simulink model "equivalent"  (R2018a)
settings: Solver=VariableStepAuto  StartTime=0.0  StopTime=10.0  RelTol=1e-3
undefined symbols (not defined in the file): DiscIntNeverNeededParam, sigbuilder_block
libraries: simulink x479
(part 4 of 10)

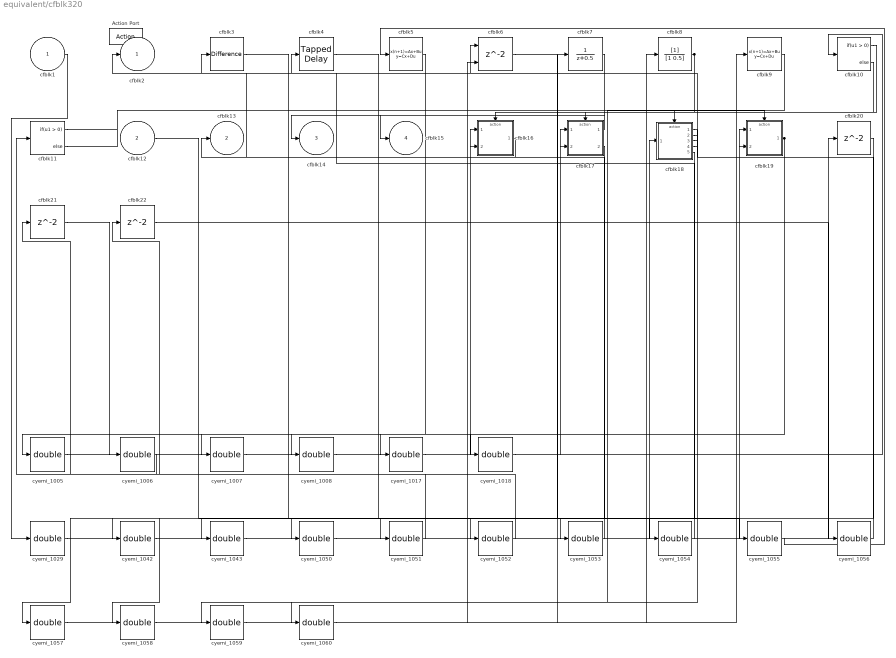
== system equivalent/cfblk320 ==
  cfblk1 : Inport
  cfblk12 : Inport  Port=2
  Action Port : ActionPort  ActionType=else
  cfblk10 : If  SampleTime=1
  cfblk11 : If  SampleTime=1
  cfblk16 : Subsystem  TreatAsAtomicUnit=on
  cfblk17 : Subsystem  TreatAsAtomicUnit=on
  cfblk18 : Subsystem  TreatAsAtomicUnit=on
  cfblk19 : Subsystem  TreatAsAtomicUnit=on
  cfblk20 : Delay
  cfblk21 : Delay
  cfblk22 : Delay
  cfblk3 : simulink/Discrete/Difference  ICPrevInput=0.0  OutMin=[]  OutMax=[]  OutDataTypeStr=Inherit: Inherit via back propagation  OutDataType=fixdt(1, 16)  OutScaling=2^-10  DoSatur=off
  cfblk4 : simulink/Discrete/Tapped Delay  vinit=0.0  samptime=-1  NumDelays=1  DelayOrder=Oldest  includeCurrent=off
  cfblk5 : DiscreteStateSpace  SampleTime=-1
  cfblk6 : Delay  ShowEnablePort=on
      settings: InputPortMap=u0,e6
  cfblk7 : DiscreteTransferFcn
  cfblk8 : DiscreteFilter
  cfblk9 : DiscreteStateSpace  SampleTime=-1
  cyemi_{1005..1008,1017..1018,1029,1042..1043,1050..1060} (20 alike) : DataTypeConversion  OutDataTypeStr=double
  cfblk2 : Outport
  cfblk13 : Outport  Port=2
  cfblk14 : Outport  Port=3
  cfblk15 : Outport  Port=4
  wires:
  cfblk8/1 -> cyemi_1007/1, cyemi_1050/1, cyemi_1060/1
  cfblk16/1(cfblk2) -> cfblk13/1
  cfblk19/1(cfblk2) -> cyemi_1005/1, cyemi_1008/1
  cfblk17/1(cfblk2) -> cfblk14/1
  cfblk18/3(cfblk14) -> cfblk2/1
  cfblk7/1 -> cfblk15/1
  cfblk10/1 -> cfblk16/Action
  cfblk10/2 -> cfblk17/Action
  cfblk11/1 -> cfblk18/Action
  cfblk11/2 -> cfblk19/Action
  cyemi_1005/1 -> cfblk10/1
  cyemi_1006/1 -> cfblk11/1
  cfblk21/1 -> cyemi_1006/1
  cyemi_1007/1 -> cfblk16/1(cfblk1)
  cyemi_1008/1 -> cfblk16/2(cfblk8)
  cyemi_1017/1 -> cfblk17/1(cfblk1)
  cfblk5/1 -> cyemi_1017/1
  cyemi_1018/1 -> cfblk17/2(cfblk10)
  cfblk18/1(cfblk2) -> cyemi_1018/1
  cyemi_1029/1 -> cfblk18/1(cfblk1)
  cfblk1/1 -> cyemi_1029/1
  cyemi_1042/1 -> cfblk19/1(cfblk1)
  cfblk20/1 -> cyemi_1042/1
  cyemi_1043/1 -> cfblk19/2(cfblk8)
  cfblk18/2(cfblk13) -> cyemi_1043/1
  cyemi_1050/1 -> cfblk20/1
  cyemi_1051/1 -> cfblk21/1
  cfblk3/1 -> cyemi_1051/1
  cyemi_1052/1 -> cfblk22/1
  cfblk4/1 -> cyemi_1052/1
  cyemi_1053/1 -> cfblk3/1
  cfblk9/1 -> cyemi_1053/1
  cyemi_1054/1 -> cfblk4/1
  cfblk6/1 -> cyemi_1054/1
  cyemi_1055/1 -> cfblk5/1
  cfblk12/1 -> cyemi_1055/1
  cyemi_1056/1 -> cfblk6/1
  cfblk22/1 -> cyemi_1056/1
  cyemi_1057/1 -> cfblk6/2
  cfblk18/5(cfblk16) -> cyemi_1057/1
  cyemi_1058/1 -> cfblk7/1
  cfblk17/2(cfblk11) -> cyemi_1058/1
  cyemi_1059/1 -> cfblk8/1
  cfblk18/4(cfblk15) -> cyemi_1059/1
  cyemi_1060/1 -> cfblk9/1

== system equivalent/cfblk321 ==
  cfblk1 : Inport
  cfblk6 : Inport  Port=2
  Action Port : ActionPort  ActionType=then
  cfblk10 : Subsystem  TreatAsAtomicUnit=on
  cfblk11 : Delay
  cfblk12 : Delay
  cfblk3 : simulink/Discrete/Transfer Fcn Real Zero  ZeroZ=0.75  ICPrevInput=0.0  DoSatur=off
      settings: SourceProductName=Simulink  SourceProductBaseCode=SL
  cfblk4 : simulink/Discrete/Transfer Fcn Lead or Lag  PoleZ=0.95  ZeroZ=0.75  ICPrevOutput=0.0  ICPrevInput=0.0  DoSatur=off
      settings: SourceProductName=Simulink  SourceProductBaseCode=SL
  cfblk5 : If  SampleTime=1
  cfblk9 : Subsystem  TreatAsAtomicUnit=on
  cyemi_{1063..1064,1075..1081} (9 alike) : DataTypeConversion  OutDataTypeStr=double
  cfblk2 : Outport
  cfblk7 : Outport  Port=2
  cfblk8 : Outport  Port=3
  wires:
  cfblk9/1(cfblk2) -> cfblk8/1, cyemi_1075/1, cyemi_1077/1
  cfblk10/3(cfblk14) -> cfblk7/1
  cfblk3/1 -> cfblk2/1
  cfblk5/1 -> cfblk9/Action
  cfblk5/2 -> cfblk10/Action
  cyemi_1063/1 -> cfblk10/1(cfblk1)
  cfblk11/1 -> cyemi_1063/1
  cyemi_1064/1 -> cfblk10/2(cfblk12)
  cfblk1/1 -> cyemi_1064/1
  cyemi_1075/1 -> cfblk11/1
  cyemi_1076/1 -> cfblk12/1
  cfblk4/1 -> cyemi_1076/1
  cyemi_1077/1 -> cfblk3/1
  cyemi_1078/1 -> cfblk4/1
  cfblk10/2(cfblk13) -> cyemi_1078/1
  cyemi_1079/1 -> cfblk5/1
  cfblk6/1 -> cyemi_1079/1
  cyemi_1080/1 -> cfblk9/1(cfblk1)
  cfblk12/1 -> cyemi_1080/1
  cyemi_1081/1 -> cfblk9/2(cfblk8)
  cfblk10/1(cfblk2) -> cyemi_1081/1

== system equivalent/cfblk322 ==
  cfblk1 : Inport
  cfblk11 : Inport  Port=2
  Action Port : ActionPort  ActionType=else
  cfblk{6,10,13..15} (5 alike) : Delay
  cfblk3 : UnitDelay  SampleTime=-1
  cfblk4 : simulink/Continuous/PID Controller (2DOF)  Controller=PID  TimeDomain=Discrete-time  SampleTime=-1  IntegratorMethod=Forward Euler  FilterMethod=Forward Euler  Form=Parallel  UseFilter=on  ControllerParametersSource=internal  P=1  I=1  D=0  N=100  b=1  c=1  InitialConditionSource=internal  InitialConditionForIntegrator=0  InitialConditionForFilter=0  ExternalReset=none  LimitOutput=off  UpperSaturationLimit=inf  LowerSaturationLimit=-inf  LinearizeAsGain=off  AntiWindupMode=none  Kb=1  TrackingMode=off  Kt=1  PParamMin=[]  PParamMax=[]  IParamMin=[]  IParamMax=[]  DParamMin=[]  DParamMax=[]  NParamMin=[]  NParamMax=[]  bParamMin=[]  bParamMax=[]  cParamMin=[]  cParamMax=[]  KbParamMin=[]  KbParamMax=[]  KtParamMin=[]  KtParamMax=[]  POutMin=[]  POutMax=[]  IOutMin=[]  IOutMax=[]  DOutMin=[]  DOutMax=[]  NOutMin=[]  NOutMax=[]  bOutMin=[]  bOutMax=[]  cOutMin=[]  cOutMax=[]  KbOutMin=[]  KbOutMax=[]  KtOutMin=[]  KtOutMax=[]  IntegratorOutMin=[]  IntegratorOutMax=[]  FilterOutMin=[]  FilterOutMax=[]  SumOutMin=[]  SumOutMax=[]  Sum1OutMin=[]  Sum1OutMax=[]  Sum2OutMin=[]  Sum2OutMax=[]  Sum3OutMin=[]  Sum3OutMax=[]  SumI1OutMin=[]  SumI1OutMax=[]  SumI2OutMin=[]  SumI2OutMax=[]  SumI3OutMin=[]  SumI3OutMax=[]  SumDOutMin=[]  SumDOutMax=[]  SaturationOutMin=[]  SaturationOutMax=[]  IntegratorContinuousStateAttributes=''  IntegratorStateMustResolveToSignalObject=off  IntegratorRTWStateStorageClass=Auto  FilterContinuousStateAttributes=''  FilterStateMustResolveToSignalObject=off  FilterRTWStateStorageClass=Auto  DifferentiatorICPrevScaledInput=0  DifferentiatorOutMin=[]  DifferentiatorOutMax=[]  FilterDiffOutCoefMin=[]  FilterDiffOutCoefMax=[]  SumDenOutMin=[]  SumDenOutMax=[]  SumNumOutMin=[]  SumNumOutMax=[]  ReciprocalOutMin=[]  ReciprocalOutMax=[]  DivideOutMin=[]  DivideOutMax=[]  TunerSelectOption=Transfer Function Based (PID Tuner App)
  cfblk5 : DiscreteZeroPole  Poles=[0 0.5]  Gain=1  SampleTime=-1
  cfblk7 : Delay  DelayLengthSource=Input port
      settings: InputPortMap=u0,p1
  cfblk8 : DiscreteTransferFcn
  cfblk9 : DiscreteZeroPole  Poles=[0 0.5]  Gain=1  SampleTime=-1
  cyemi_{1090..1102} (13 alike) : DataTypeConversion  OutDataTypeStr=double
  cfblk2 : Outport
  cfblk12 : Outport  Port=2
  wires:
  cfblk3/1 -> cfblk2/1
  cfblk8/1 -> cfblk12/1, cyemi_1100/1
  cfblk9/1 -> cyemi_1091/1, cyemi_1098/1
  cyemi_1090/1 -> cfblk10/1
  cfblk6/1 -> cyemi_1090/1
  cyemi_1091/1 -> cfblk13/1
  cyemi_1092/1 -> cfblk14/1
  cfblk10/1 -> cyemi_1092/1
  cyemi_1093/1 -> cfblk15/1
  cfblk7/1 -> cyemi_1093/1
  cyemi_1094/1 -> cfblk3/1
  cfblk1/1 -> cyemi_1094/1
  cyemi_1095/1 -> cfblk4/1
  cfblk13/1 -> cyemi_1095/1
  cyemi_1096/1 -> cfblk4/2
  cfblk14/1 -> cyemi_1096/1
  cyemi_1097/1 -> cfblk5/1
  cfblk15/1 -> cyemi_1097/1
  cyemi_1098/1 -> cfblk6/1
  cyemi_1099/1 -> cfblk7/1
  cfblk11/1 -> cyemi_1099/1
  cyemi_1100/1 -> cfblk7/2
  cyemi_1101/1 -> cfblk8/1
  cfblk5/1 -> cyemi_1101/1
  cyemi_1102/1 -> cfblk9/1
  cfblk4/1 -> cyemi_1102/1

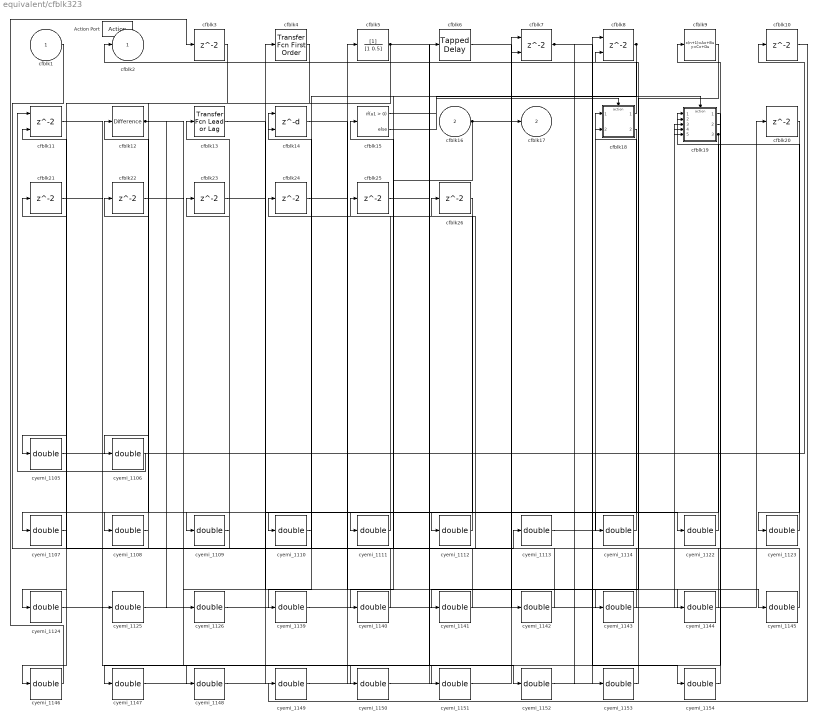
== system equivalent/cfblk323 ==
  cfblk1 : Inport
  cfblk16 : Inport  Port=2
  Action Port : ActionPort  ActionType=then
  cfblk{3,10,20..26} (9 alike) : Delay
  cfblk11 : Delay  ShowEnablePort=on
      settings: InputPortMap=u0,e6
  cfblk12 : simulink/Discrete/Difference  ICPrevInput=0.0  OutMin=[]  OutMax=[]  OutDataTypeStr=Inherit: Inherit via back propagation  OutDataType=fixdt(1, 16)  OutScaling=2^-10  DoSatur=off
  cfblk13 : simulink/Discrete/Transfer Fcn Lead or Lag  PoleZ=0.95  ZeroZ=0.75  ICPrevOutput=0.0  ICPrevInput=0.0  DoSatur=off
      settings: SourceProductName=Simulink  SourceProductBaseCode=SL
  cfblk14 : Delay  DelayLengthSource=Input port
      settings: InputPortMap=u0,p1
  cfblk15 : If  SampleTime=1
  cfblk18 : Subsystem  TreatAsAtomicUnit=on
  cfblk19 : Subsystem  TreatAsAtomicUnit=on
  cfblk4 : simulink/Discrete/Transfer Fcn First Order  PoleZ=0.95  ICPrevOutput=0.0  DoSatur=off
      settings: SourceProductName=Simulink
  cfblk5 : DiscreteFilter
  cfblk6 : simulink/Discrete/Tapped Delay  vinit=0.0  samptime=-1  NumDelays=1  DelayOrder=Oldest  includeCurrent=off
  cfblk7 : Delay  ShowEnablePort=on
      settings: InputPortMap=u0,e6
  cfblk8 : Delay  ShowEnablePort=on
      settings: InputPortMap=u0,e6
  cfblk9 : DiscreteStateSpace  SampleTime=-1
  cyemi_{1105..1114,1122..1126,1139..1154} (31 alike) : DataTypeConversion  OutDataTypeStr=double
  cfblk2 : Outport
  cfblk17 : Outport  Port=2
  wires:
  cfblk16/1 -> cfblk17/1, cyemi_1111/1
  cfblk5/1 -> cyemi_1107/1, cyemi_1152/1
  cfblk12/1 -> cyemi_1106/1, cyemi_1126/1, cyemi_1145/1
  cfblk18/1(cfblk2) -> cfblk2/1
  cfblk8/1 -> cyemi_1139/1, cyemi_1140/1
  cfblk7/1 -> cyemi_1153/1, cyemi_1154/1
  cfblk19/3(cfblk16) -> cyemi_1109/1, cyemi_1110/1
  cfblk15/1 -> cfblk18/Action
  cfblk15/2 -> cfblk19/Action
  cyemi_1105/1 -> cfblk10/1
  cfblk4/1 -> cyemi_1105/1
  cyemi_1106/1 -> cfblk11/1
  cyemi_1107/1 -> cfblk11/2
  cyemi_1108/1 -> cfblk12/1
  cfblk3/1 -> cyemi_1108/1
  cyemi_1109/1 -> cfblk13/1
  cyemi_1110/1 -> cfblk14/1
  cyemi_1111/1 -> cfblk14/2
  cyemi_1112/1 -> cfblk15/1
  cfblk23/1 -> cyemi_1112/1
  cyemi_1113/1 -> cfblk18/1(cfblk1)
  cfblk1/1 -> cyemi_1113/1
  cyemi_1114/1 -> cfblk18/2(cfblk9)
  cfblk25/1 -> cyemi_1114/1
  cyemi_1122/1 -> cfblk19/1(cfblk1)
  cfblk24/1 -> cyemi_1122/1
  cyemi_1123/1 -> cfblk19/2(cfblk11)
  cfblk20/1 -> cyemi_1123/1
  cyemi_1124/1 -> cfblk19/3(cfblk12)
  cfblk18/2(cfblk10) -> cyemi_1124/1
  cyemi_1125/1 -> cfblk19/4(cfblk13)
  cfblk21/1 -> cyemi_1125/1
  cyemi_1126/1 -> cfblk19/5(cfblk14)
  cyemi_1139/1 -> cfblk20/1
  cyemi_1140/1 -> cfblk21/1
  cyemi_1141/1 -> cfblk22/1
  cfblk9/1 -> cyemi_1141/1
  cyemi_1142/1 -> cfblk23/1
  cfblk6/1 -> cyemi_1142/1
  cyemi_1143/1 -> cfblk24/1
  cfblk14/1 -> cyemi_1143/1
  cyemi_1144/1 -> cfblk25/1
  cfblk13/1 -> cyemi_1144/1
  cyemi_1145/1 -> cfblk26/1
  cyemi_1146/1 -> cfblk3/1
  cfblk26/1 -> cyemi_1146/1
  cyemi_1147/1 -> cfblk4/1
  cfblk19/2(cfblk15) -> cyemi_1147/1
  cyemi_1148/1 -> cfblk5/1
  cfblk19/1(cfblk2) -> cyemi_1148/1
  cyemi_1149/1 -> cfblk6/1
  cfblk10/1 -> cyemi_1149/1
  cyemi_1150/1 -> cfblk7/1
  cfblk11/1 -> cyemi_1150/1
  cyemi_1151/1 -> cfblk7/2
  cfblk22/1 -> cyemi_1151/1
  cyemi_1152/1 -> cfblk8/1
  cyemi_1153/1 -> cfblk8/2
  cyemi_1154/1 -> cfblk9/1

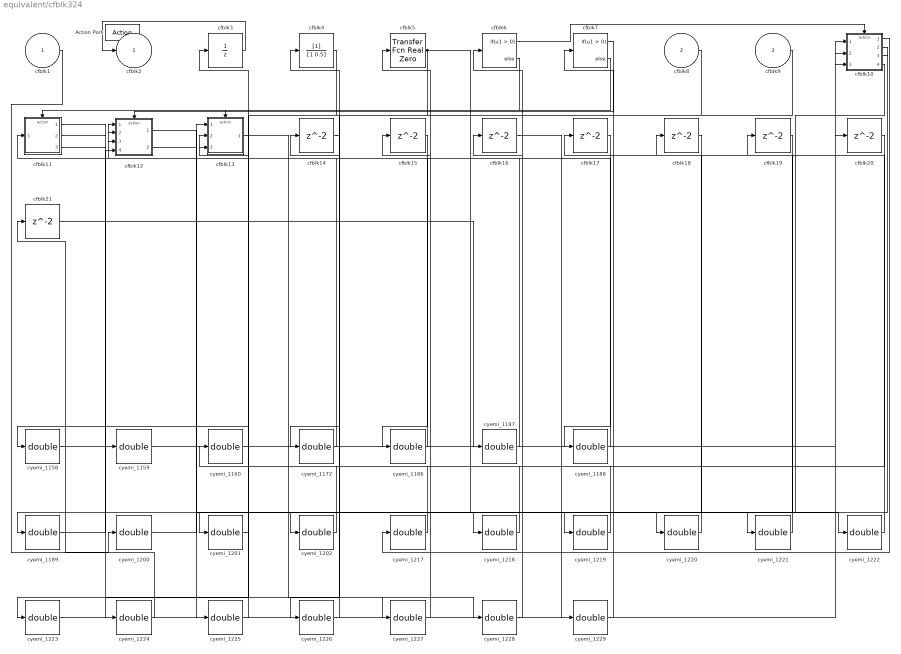
== system equivalent/cfblk324 ==
  cfblk1 : Inport
  cfblk8 : Inport  Port=2
  cfblk9 : Inport  Port=3
  Action Port : ActionPort  ActionType=else
  cfblk10 : Subsystem  TreatAsAtomicUnit=on
  cfblk11 : Subsystem  TreatAsAtomicUnit=on
  cfblk12 : Subsystem  TreatAsAtomicUnit=on
  cfblk13 : Subsystem  TreatAsAtomicUnit=on
  cfblk{14..21} (8 alike) : Delay
  cfblk3 : UnitDelay  SampleTime=-1
  cfblk4 : DiscreteFilter
  cfblk5 : simulink/Discrete/Transfer Fcn Real Zero  ZeroZ=0.75  ICPrevInput=0.0  DoSatur=off
      settings: SourceProductName=Simulink  SourceProductBaseCode=SL
  cfblk6 : If  SampleTime=1
  cfblk7 : If  SampleTime=1
  cyemi_{1158..1160,1172,1186..1189,1200..1202,1217..1229} (24 alike) : DataTypeConversion  OutDataTypeStr=double
  cfblk2 : Outport
  wires:
  cfblk3/1 -> cfblk2/1
  cfblk5/1 -> cyemi_1222/1, cyemi_1223/1
  cfblk6/1 -> cfblk10/Action
  cfblk6/2 -> cfblk11/Action
  cfblk7/1 -> cfblk12/Action
  cfblk7/2 -> cfblk13/Action
  cyemi_1158/1 -> cfblk10/1(cfblk1)
  cfblk4/1 -> cyemi_1158/1
  cyemi_1159/1 -> cfblk10/2(cfblk12)
  cfblk11/2(cfblk10) -> cyemi_1159/1
  cyemi_1160/1 -> cfblk10/3(cfblk13)
  cfblk20/1 -> cyemi_1160/1
  cyemi_1172/1 -> cfblk11/1(cfblk1)
  cfblk9/1 -> cyemi_1172/1
  cyemi_1186/1 -> cfblk12/1(cfblk1)
  cfblk15/1 -> cyemi_1186/1
  cyemi_1187/1 -> cfblk12/2(cfblk12)
  cfblk21/1 -> cyemi_1187/1
  cyemi_1188/1 -> cfblk12/3(cfblk13)
  cfblk17/1 -> cyemi_1188/1
  cyemi_1189/1 -> cfblk12/4(cfblk14)
  cfblk18/1 -> cyemi_1189/1
  cyemi_1200/1 -> cfblk13/1(cfblk1)
  cfblk1/1 -> cyemi_1200/1
  cyemi_1201/1 -> cfblk13/2(cfblk13)
  cfblk19/1 -> cyemi_1201/1
  cyemi_1202/1 -> cfblk13/3(cfblk14)
  cfblk14/1 -> cyemi_1202/1
  cyemi_1217/1 -> cfblk14/1
  cfblk10/1(cfblk2) -> cyemi_1217/1
  cyemi_1218/1 -> cfblk15/1
  cfblk10/2(cfblk14) -> cyemi_1218/1
  cyemi_1219/1 -> cfblk16/1
  cfblk12/1(cfblk2) -> cyemi_1219/1
  cyemi_1220/1 -> cfblk17/1
  cfblk10/3(cfblk15) -> cyemi_1220/1
  cyemi_1221/1 -> cfblk18/1
  cfblk10/4(cfblk16) -> cyemi_1221/1
  cyemi_1222/1 -> cfblk19/1
  cyemi_1223/1 -> cfblk20/1
  cyemi_1224/1 -> cfblk21/1
  cfblk11/3(cfblk11) -> cyemi_1224/1
  cyemi_1225/1 -> cfblk3/1
  cfblk12/2(cfblk15) -> cyemi_1225/1
  cyemi_1226/1 -> cfblk4/1
  cfblk8/1 -> cyemi_1226/1
  cyemi_1227/1 -> cfblk5/1
  cfblk11/1(cfblk2) -> cyemi_1227/1
  cyemi_1228/1 -> cfblk6/1
  cfblk13/1(cfblk2) -> cyemi_1228/1
  cyemi_1229/1 -> cfblk7/1
  cfblk16/1 -> cyemi_1229/1

== system equivalent/cfblk325 ==
  cfblk1 : Inport
  cfblk6 : Inport  Port=2
  Action Port : ActionPort  ActionType=then
  cfblk3 : Delay
  cfblk4 : simulink/Continuous/PID Controller (2DOF)  Controller=PID  TimeDomain=Discrete-time  SampleTime=-1  IntegratorMethod=Forward Euler  FilterMethod=Forward Euler  Form=Parallel  UseFilter=on  ControllerParametersSource=internal  P=1  I=1  D=0  N=100  b=1  c=1  InitialConditionSource=internal  InitialConditionForIntegrator=0  InitialConditionForFilter=0  ExternalReset=none  LimitOutput=off  UpperSaturationLimit=inf  LowerSaturationLimit=-inf  LinearizeAsGain=off  AntiWindupMode=none  Kb=1  TrackingMode=off  Kt=1  PParamMin=[]  PParamMax=[]  IParamMin=[]  IParamMax=[]  DParamMin=[]  DParamMax=[]  NParamMin=[]  NParamMax=[]  bParamMin=[]  bParamMax=[]  cParamMin=[]  cParamMax=[]  KbParamMin=[]  KbParamMax=[]  KtParamMin=[]  KtParamMax=[]  POutMin=[]  POutMax=[]  IOutMin=[]  IOutMax=[]  DOutMin=[]  DOutMax=[]  NOutMin=[]  NOutMax=[]  bOutMin=[]  bOutMax=[]  cOutMin=[]  cOutMax=[]  KbOutMin=[]  KbOutMax=[]  KtOutMin=[]  KtOutMax=[]  IntegratorOutMin=[]  IntegratorOutMax=[]  FilterOutMin=[]  FilterOutMax=[]  SumOutMin=[]  SumOutMax=[]  Sum1OutMin=[]  Sum1OutMax=[]  Sum2OutMin=[]  Sum2OutMax=[]  Sum3OutMin=[]  Sum3OutMax=[]  SumI1OutMin=[]  SumI1OutMax=[]  SumI2OutMin=[]  SumI2OutMax=[]  SumI3OutMin=[]  SumI3OutMax=[]  SumDOutMin=[]  SumDOutMax=[]  SaturationOutMin=[]  SaturationOutMax=[]  IntegratorContinuousStateAttributes=''  IntegratorStateMustResolveToSignalObject=off  IntegratorRTWStateStorageClass=Auto  FilterContinuousStateAttributes=''  FilterStateMustResolveToSignalObject=off  FilterRTWStateStorageClass=Auto  DifferentiatorICPrevScaledInput=0  DifferentiatorOutMin=[]  DifferentiatorOutMax=[]  FilterDiffOutCoefMin=[]  FilterDiffOutCoefMax=[]  SumDenOutMin=[]  SumDenOutMax=[]  SumNumOutMin=[]  SumNumOutMax=[]  ReciprocalOutMin=[]  ReciprocalOutMax=[]  DivideOutMin=[]  DivideOutMax=[]  TunerSelectOption=Transfer Function Based (PID Tuner App)
  cfblk5 : simulink/Discrete/Tapped Delay  vinit=0.0  samptime=-1  NumDelays=1  DelayOrder=Oldest  includeCurrent=off
  cyemi_{1232..1235} (4 alike) : DataTypeConversion  OutDataTypeStr=double
  cfblk2 : Outport
  cfblk7 : Outport  Port=2
  wires:
  cfblk3/1 -> cfblk2/1, cyemi_1234/1
  cfblk4/1 -> cfblk7/1
  cyemi_1232/1 -> cfblk3/1
  cfblk1/1 -> cyemi_1232/1
  cyemi_1233/1 -> cfblk4/1
  cfblk5/1 -> cyemi_1233/1
  cyemi_1234/1 -> cfblk4/2
  cyemi_1235/1 -> cfblk5/1
  cfblk6/1 -> cyemi_1235/1

== system equivalent/cfblk326 ==
  cfblk1 : Inport
  cfblk6 : Inport  Port=2
  cfblk7 : Inport  Port=3
  cfblk8 : Inport  Port=4
  cfblk9 : Inport  Port=5
  Action Port : ActionPort  ActionType=else
  cfblk11 : Delay
  cfblk3 : Delay  DelayLengthSource=Input port
      settings: InputPortMap=u0,p1
  cfblk4 : DiscreteFir
  cfblk5 : DiscreteZeroPole  Poles=[0 0.5]  Gain=1  SampleTime=-1
  cyemi_{1241..1245} (5 alike) : DataTypeConversion  OutDataTypeStr=double
  cfblk2 : Outport
  cfblk10 : Outport  Port=2
  wires:
  cfblk8/1 -> cfblk2/1
  cfblk7/1 -> cfblk10/1
  cyemi_1241/1 -> cfblk11/1
  cfblk4/1 -> cyemi_1241/1
  cyemi_1242/1 -> cfblk3/1
  cfblk1/1 -> cyemi_1242/1
  cyemi_1243/1 -> cfblk3/2
  cfblk11/1 -> cyemi_1243/1
  cyemi_1244/1 -> cfblk4/1
  cfblk5/1 -> cyemi_1244/1
  cyemi_1245/1 -> cfblk5/1
  cfblk3/1 -> cyemi_1245/1

== system equivalent/cfblk327 ==
  cfblk1 : Inport
  cfblk11 : Inport  Port=2
  Action Port : ActionPort  ActionType=then
  cfblk10 : If  SampleTime=1
  cfblk12 : Subsystem  TreatAsAtomicUnit=on
  cfblk13 : Subsystem  TreatAsAtomicUnit=on
  cfblk14 : Delay
  cfblk15 : Delay
  cfblk16 : Delay
  cfblk3 : DiscreteZeroPole  Poles=[0 0.5]  Gain=1  SampleTime=-1
  cfblk4 : DiscreteStateSpace  SampleTime=-1
  cfblk5 : DiscreteIntegrator  SampleTime=-1  ICPrevOutput=DiscIntNeverNeededParam  ICPrevScaledInput=DiscIntNeverNeededParam
  cfblk6 : simulink/Discrete/Transfer Fcn First Order  PoleZ=0.95  ICPrevOutput=0.0  DoSatur=off
      settings: SourceProductName=Simulink
  cfblk7 : DiscreteIntegrator  SampleTime=-1  ICPrevOutput=DiscIntNeverNeededParam  ICPrevScaledInput=DiscIntNeverNeededParam
  cfblk8 : Delay  ShowEnablePort=on
      settings: InputPortMap=u0,e6
  cfblk9 : simulink/Continuous/PID Controller  Controller=PID  TimeDomain=Discrete-time  SampleTime=-1  IntegratorMethod=Forward Euler  FilterMethod=Forward Euler  Form=Parallel  UseFilter=on  ControllerParametersSource=internal  P=1  I=1  D=0  N=100  InitialConditionSource=internal  InitialConditionForIntegrator=0  InitialConditionForFilter=0  ExternalReset=none  LimitOutput=off  UpperSaturationLimit=inf  LowerSaturationLimit=-inf  LinearizeAsGain=off  AntiWindupMode=none  Kb=1  TrackingMode=off  Kt=1  PParamMin=[]  PParamMax=[]  IParamMin=[]  IParamMax=[]  DParamMin=[]  DParamMax=[]  NParamMin=[]  NParamMax=[]  KbParamMin=[]  KbParamMax=[]  KtParamMin=[]  KtParamMax=[]  POutMin=[]  POutMax=[]  IOutMin=[]  IOutMax=[]  DOutMin=[]  DOutMax=[]  NOutMin=[]  NOutMax=[]  KbOutMin=[]  KbOutMax=[]  KtOutMin=[]  KtOutMax=[]  IntegratorOutMin=[]  IntegratorOutMax=[]  FilterOutMin=[]  FilterOutMax=[]  SumOutMin=[]  SumOutMax=[]  SumI1OutMin=[]  SumI1OutMax=[]  SumI2OutMin=[]  SumI2OutMax=[]  SumI3OutMin=[]  SumI3OutMax=[]  SumDOutMin=[]  SumDOutMax=[]  SaturationOutMin=[]  SaturationOutMax=[]  IntegratorContinuousStateAttributes=''  IntegratorStateMustResolveToSignalObject=off  IntegratorRTWStateStorageClass=Auto  FilterContinuousStateAttributes=''  FilterStateMustResolveToSignalObject=off  FilterRTWStateStorageClass=Auto  DifferentiatorICPrevScaledInput=0  DifferentiatorOutMin=[]  DifferentiatorOutMax=[]  FilterDiffOutCoefMin=[]  FilterDiffOutCoefMax=[]  SumDenOutMin=[]  SumDenOutMax=[]  SumNumOutMin=[]  SumNumOutMax=[]  ReciprocalOutMin=[]  ReciprocalOutMax=[]  DivideOutMin=[]  DivideOutMax=[]  TunerSelectOption=Transfer Function Based (PID Tuner App)
  cyemi_{1248..1251,1261,1271..1281} (16 alike) : DataTypeConversion  OutDataTypeStr=double
  cfblk2 : Outport
  wires:
  cfblk4/1 -> cfblk2/1
  cfblk1/1 -> cyemi_1251/1, cyemi_1274/1
  cfblk12/2(cfblk13) -> cyemi_1273/1, cyemi_1280/1
  cfblk10/1 -> cfblk12/Action
  cfblk10/2 -> cfblk13/Action
  cyemi_1248/1 -> cfblk10/1
  cfblk16/1 -> cyemi_1248/1
  cyemi_1249/1 -> cfblk12/1(cfblk1)
  cfblk6/1 -> cyemi_1249/1
  cyemi_1250/1 -> cfblk12/2(cfblk11)
  cfblk11/1 -> cyemi_1250/1
  cyemi_1251/1 -> cfblk12/3(cfblk12)
  cyemi_1261/1 -> cfblk13/1(cfblk1)
  cfblk14/1 -> cyemi_1261/1
  cyemi_1271/1 -> cfblk14/1
  cfblk5/1 -> cyemi_1271/1
  cyemi_1272/1 -> cfblk15/1
  cfblk13/1(cfblk2) -> cyemi_1272/1
  cyemi_1273/1 -> cfblk16/1
  cyemi_1274/1 -> cfblk3/1
  cyemi_1275/1 -> cfblk4/1
  cfblk12/1(cfblk2) -> cyemi_1275/1
  cyemi_1276/1 -> cfblk5/1
  cfblk7/1 -> cyemi_1276/1
  cyemi_1277/1 -> cfblk6/1
  cfblk3/1 -> cyemi_1277/1
  cyemi_1278/1 -> cfblk7/1
  cfblk9/1 -> cyemi_1278/1
  cyemi_1279/1 -> cfblk8/1
  cfblk15/1 -> cyemi_1279/1
  cyemi_1280/1 -> cfblk8/2
  cyemi_1281/1 -> cfblk9/1
  cfblk8/1 -> cyemi_1281/1

== system equivalent/cfblk328 ==
  cfblk1 : Inport
  cfblk7 : Inport  Port=2
  cfblk8 : Inport  Port=3
  Action Port : ActionPort  ActionType=else
  cfblk10 : Delay
  cfblk3 : simulink/Continuous/PID Controller  Controller=PID  TimeDomain=Discrete-time  SampleTime=-1  IntegratorMethod=Forward Euler  FilterMethod=Forward Euler  Form=Parallel  UseFilter=on  ControllerParametersSource=internal  P=1  I=1  D=0  N=100  InitialConditionSource=internal  InitialConditionForIntegrator=0  InitialConditionForFilter=0  ExternalReset=none  LimitOutput=off  UpperSaturationLimit=inf  LowerSaturationLimit=-inf  LinearizeAsGain=off  AntiWindupMode=none  Kb=1  TrackingMode=off  Kt=1  PParamMin=[]  PParamMax=[]  IParamMin=[]  IParamMax=[]  DParamMin=[]  DParamMax=[]  NParamMin=[]  NParamMax=[]  KbParamMin=[]  KbParamMax=[]  KtParamMin=[]  KtParamMax=[]  POutMin=[]  POutMax=[]  IOutMin=[]  IOutMax=[]  DOutMin=[]  DOutMax=[]  NOutMin=[]  NOutMax=[]  KbOutMin=[]  KbOutMax=[]  KtOutMin=[]  KtOutMax=[]  IntegratorOutMin=[]  IntegratorOutMax=[]  FilterOutMin=[]  FilterOutMax=[]  SumOutMin=[]  SumOutMax=[]  SumI1OutMin=[]  SumI1OutMax=[]  SumI2OutMin=[]  SumI2OutMax=[]  SumI3OutMin=[]  SumI3OutMax=[]  SumDOutMin=[]  SumDOutMax=[]  SaturationOutMin=[]  SaturationOutMax=[]  IntegratorContinuousStateAttributes=''  IntegratorStateMustResolveToSignalObject=off  IntegratorRTWStateStorageClass=Auto  FilterContinuousStateAttributes=''  FilterStateMustResolveToSignalObject=off  FilterRTWStateStorageClass=Auto  DifferentiatorICPrevScaledInput=0  DifferentiatorOutMin=[]  DifferentiatorOutMax=[]  FilterDiffOutCoefMin=[]  FilterDiffOutCoefMax=[]  SumDenOutMin=[]  SumDenOutMax=[]  SumNumOutMin=[]  SumNumOutMax=[]  ReciprocalOutMin=[]  ReciprocalOutMax=[]  DivideOutMin=[]  DivideOutMax=[]  TunerSelectOption=Transfer Function Based (PID Tuner App)
  cfblk4 : DiscreteTransferFcn
  cfblk5 : DiscreteTransferFcn
  cfblk6 : simulink/Continuous/PID Controller (2DOF)  Controller=PID  TimeDomain=Discrete-time  SampleTime=-1  IntegratorMethod=Forward Euler  FilterMethod=Forward Euler  Form=Parallel  UseFilter=on  ControllerParametersSource=internal  P=1  I=1  D=0  N=100  b=1  c=1  InitialConditionSource=internal  InitialConditionForIntegrator=0  InitialConditionForFilter=0  ExternalReset=none  LimitOutput=off  UpperSaturationLimit=inf  LowerSaturationLimit=-inf  LinearizeAsGain=off  AntiWindupMode=none  Kb=1  TrackingMode=off  Kt=1  PParamMin=[]  PParamMax=[]  IParamMin=[]  IParamMax=[]  DParamMin=[]  DParamMax=[]  NParamMin=[]  NParamMax=[]  bParamMin=[]  bParamMax=[]  cParamMin=[]  cParamMax=[]  KbParamMin=[]  KbParamMax=[]  KtParamMin=[]  KtParamMax=[]  POutMin=[]  POutMax=[]  IOutMin=[]  IOutMax=[]  DOutMin=[]  DOutMax=[]  NOutMin=[]  NOutMax=[]  bOutMin=[]  bOutMax=[]  cOutMin=[]  cOutMax=[]  KbOutMin=[]  KbOutMax=[]  KtOutMin=[]  KtOutMax=[]  IntegratorOutMin=[]  IntegratorOutMax=[]  FilterOutMin=[]  FilterOutMax=[]  SumOutMin=[]  SumOutMax=[]  Sum1OutMin=[]  Sum1OutMax=[]  Sum2OutMin=[]  Sum2OutMax=[]  Sum3OutMin=[]  Sum3OutMax=[]  SumI1OutMin=[]  SumI1OutMax=[]  SumI2OutMin=[]  SumI2OutMax=[]  SumI3OutMin=[]  SumI3OutMax=[]  SumDOutMin=[]  SumDOutMax=[]  SaturationOutMin=[]  SaturationOutMax=[]  IntegratorContinuousStateAttributes=''  IntegratorStateMustResolveToSignalObject=off  IntegratorRTWStateStorageClass=Auto  FilterContinuousStateAttributes=''  FilterStateMustResolveToSignalObject=off  FilterRTWStateStorageClass=Auto  DifferentiatorICPrevScaledInput=0  DifferentiatorOutMin=[]  DifferentiatorOutMax=[]  FilterDiffOutCoefMin=[]  FilterDiffOutCoefMax=[]  SumDenOutMin=[]  SumDenOutMax=[]  SumNumOutMin=[]  SumNumOutMax=[]  ReciprocalOutMin=[]  ReciprocalOutMax=[]  DivideOutMin=[]  DivideOutMax=[]  TunerSelectOption=Transfer Function Based (PID Tuner App)
  cyemi_{1285..1290} (6 alike) : DataTypeConversion  OutDataTypeStr=double
  cfblk2 : Outport
  cfblk9 : Outport  Port=2
  wires:
  cfblk5/1 -> cfblk9/1
  cfblk4/1 -> cfblk2/1
  cyemi_1285/1 -> cfblk10/1
  cfblk6/1 -> cyemi_1285/1
  cyemi_1286/1 -> cfblk3/1
  cfblk10/1 -> cyemi_1286/1
  cyemi_1287/1 -> cfblk4/1
  cfblk7/1 -> cyemi_1287/1
  cyemi_1288/1 -> cfblk5/1
  cfblk1/1 -> cyemi_1288/1
  cyemi_1289/1 -> cfblk6/1
  cfblk8/1 -> cyemi_1289/1
  cyemi_1290/1 -> cfblk6/2
  cfblk3/1 -> cyemi_1290/1

== system equivalent/cfblk329 ==
  cfblk1 : Inport
  cfblk10 : Inport  Port=2
  Action Port : ActionPort  ActionType=then
  cfblk15 : Delay
  cfblk3 : simulink/Continuous/PID Controller (2DOF)  Controller=PID  TimeDomain=Discrete-time  SampleTime=-1  IntegratorMethod=Forward Euler  FilterMethod=Forward Euler  Form=Parallel  UseFilter=on  ControllerParametersSource=internal  P=1  I=1  D=0  N=100  b=1  c=1  InitialConditionSource=internal  InitialConditionForIntegrator=0  InitialConditionForFilter=0  ExternalReset=none  LimitOutput=off  UpperSaturationLimit=inf  LowerSaturationLimit=-inf  LinearizeAsGain=off  AntiWindupMode=none  Kb=1  TrackingMode=off  Kt=1  PParamMin=[]  PParamMax=[]  IParamMin=[]  IParamMax=[]  DParamMin=[]  DParamMax=[]  NParamMin=[]  NParamMax=[]  bParamMin=[]  bParamMax=[]  cParamMin=[]  cParamMax=[]  KbParamMin=[]  KbParamMax=[]  KtParamMin=[]  KtParamMax=[]  POutMin=[]  POutMax=[]  IOutMin=[]  IOutMax=[]  DOutMin=[]  DOutMax=[]  NOutMin=[]  NOutMax=[]  bOutMin=[]  bOutMax=[]  cOutMin=[]  cOutMax=[]  KbOutMin=[]  KbOutMax=[]  KtOutMin=[]  KtOutMax=[]  IntegratorOutMin=[]  IntegratorOutMax=[]  FilterOutMin=[]  FilterOutMax=[]  SumOutMin=[]  SumOutMax=[]  Sum1OutMin=[]  Sum1OutMax=[]  Sum2OutMin=[]  Sum2OutMax=[]  Sum3OutMin=[]  Sum3OutMax=[]  SumI1OutMin=[]  SumI1OutMax=[]  SumI2OutMin=[]  SumI2OutMax=[]  SumI3OutMin=[]  SumI3OutMax=[]  SumDOutMin=[]  SumDOutMax=[]  SaturationOutMin=[]  SaturationOutMax=[]  IntegratorContinuousStateAttributes=''  IntegratorStateMustResolveToSignalObject=off  IntegratorRTWStateStorageClass=Auto  FilterContinuousStateAttributes=''  FilterStateMustResolveToSignalObject=off  FilterRTWStateStorageClass=Auto  DifferentiatorICPrevScaledInput=0  DifferentiatorOutMin=[]  DifferentiatorOutMax=[]  FilterDiffOutCoefMin=[]  FilterDiffOutCoefMax=[]  SumDenOutMin=[]  SumDenOutMax=[]  SumNumOutMin=[]  SumNumOutMax=[]  ReciprocalOutMin=[]  ReciprocalOutMax=[]  DivideOutMin=[]  DivideOutMax=[]  TunerSelectOption=Transfer Function Based (PID Tuner App)
  cfblk4 : DiscreteTransferFcn
  cfblk5 : DiscreteTransferFcn
  cfblk6 : DiscreteFir
  cfblk7 : simulink/Discrete/Transfer Fcn First Order  PoleZ=0.95  ICPrevOutput=0.0  DoSatur=off
      settings: SourceProductName=Simulink
  cfblk8 : DiscreteTransferFcn
  cfblk9 : simulink/Discrete/Transfer Fcn First Order  PoleZ=0.95  ICPrevOutput=0.0  DoSatur=off
      settings: SourceProductName=Simulink
  cyemi_{1293..1301} (9 alike) : DataTypeConversion  OutDataTypeStr=double
  cfblk2 : Outport
  cfblk11 : Outport  Port=2
  cfblk12 : Outport  Port=3
  cfblk13 : Outport  Port=4
  cfblk14 : Outport  Port=5
  wires:
  cfblk7/1 -> cfblk2/1, cyemi_1301/1
  cfblk8/1 -> cfblk14/1, cfblk11/1, cyemi_1293/1
  cfblk1/1 -> cfblk12/1, cyemi_1298/1
  cfblk10/1 -> cfblk13/1
  cyemi_1293/1 -> cfblk15/1
  cyemi_1294/1 -> cfblk3/1
  cfblk15/1 -> cyemi_1294/1
  cyemi_1295/1 -> cfblk3/2
  cfblk4/1 -> cyemi_1295/1
  cyemi_1296/1 -> cfblk4/1
  cfblk6/1 -> cyemi_1296/1
  cyemi_1297/1 -> cfblk5/1
  cfblk9/1 -> cyemi_1297/1
  cyemi_1298/1 -> cfblk6/1
  cyemi_1299/1 -> cfblk7/1
  cfblk3/1 -> cyemi_1299/1
  cyemi_1300/1 -> cfblk8/1
  cfblk5/1 -> cyemi_1300/1
  cyemi_1301/1 -> cfblk9/1

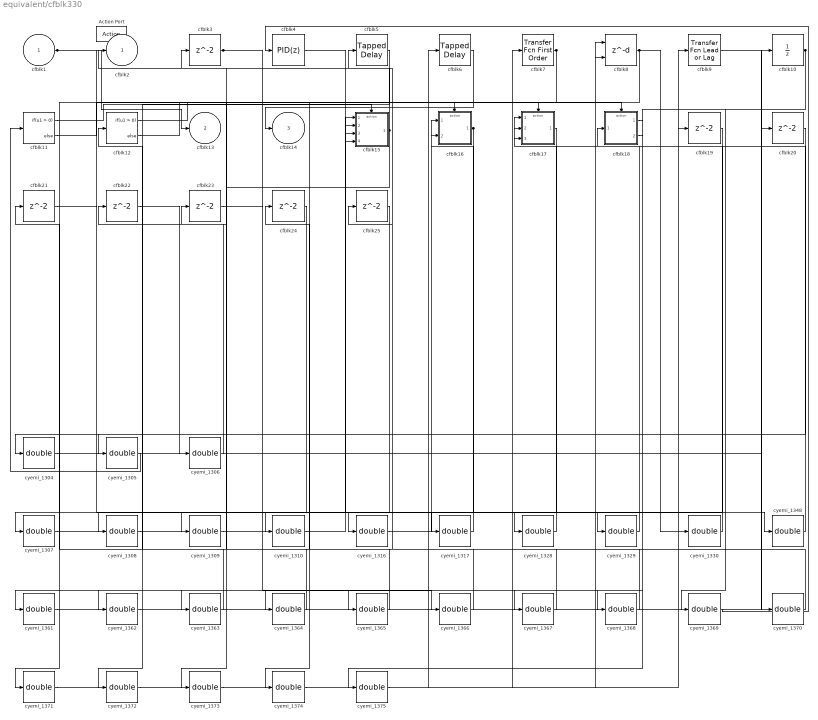
== system equivalent/cfblk330 ==
  cfblk1 : Inport
  Action Port : ActionPort  ActionType=else
  cfblk10 : UnitDelay  SampleTime=-1
  cfblk11 : If  SampleTime=1
  cfblk12 : If  SampleTime=1
  cfblk15 : Subsystem  TreatAsAtomicUnit=on
  cfblk16 : Subsystem  TreatAsAtomicUnit=on
  cfblk17 : Subsystem  TreatAsAtomicUnit=on
  cfblk18 : Subsystem  TreatAsAtomicUnit=on
  cfblk{3,19..25} (8 alike) : Delay
  cfblk4 : simulink/Continuous/PID Controller  Controller=PID  TimeDomain=Discrete-time  SampleTime=-1  IntegratorMethod=Forward Euler  FilterMethod=Forward Euler  Form=Parallel  UseFilter=on  ControllerParametersSource=internal  P=1  I=1  D=0  N=100  InitialConditionSource=internal  InitialConditionForIntegrator=0  InitialConditionForFilter=0  ExternalReset=none  LimitOutput=off  UpperSaturationLimit=inf  LowerSaturationLimit=-inf  LinearizeAsGain=off  AntiWindupMode=none  Kb=1  TrackingMode=off  Kt=1  PParamMin=[]  PParamMax=[]  IParamMin=[]  IParamMax=[]  DParamMin=[]  DParamMax=[]  NParamMin=[]  NParamMax=[]  KbParamMin=[]  KbParamMax=[]  KtParamMin=[]  KtParamMax=[]  POutMin=[]  POutMax=[]  IOutMin=[]  IOutMax=[]  DOutMin=[]  DOutMax=[]  NOutMin=[]  NOutMax=[]  KbOutMin=[]  KbOutMax=[]  KtOutMin=[]  KtOutMax=[]  IntegratorOutMin=[]  IntegratorOutMax=[]  FilterOutMin=[]  FilterOutMax=[]  SumOutMin=[]  SumOutMax=[]  SumI1OutMin=[]  SumI1OutMax=[]  SumI2OutMin=[]  SumI2OutMax=[]  SumI3OutMin=[]  SumI3OutMax=[]  SumDOutMin=[]  SumDOutMax=[]  SaturationOutMin=[]  SaturationOutMax=[]  IntegratorContinuousStateAttributes=''  IntegratorStateMustResolveToSignalObject=off  IntegratorRTWStateStorageClass=Auto  FilterContinuousStateAttributes=''  FilterStateMustResolveToSignalObject=off  FilterRTWStateStorageClass=Auto  DifferentiatorICPrevScaledInput=0  DifferentiatorOutMin=[]  DifferentiatorOutMax=[]  FilterDiffOutCoefMin=[]  FilterDiffOutCoefMax=[]  SumDenOutMin=[]  SumDenOutMax=[]  SumNumOutMin=[]  SumNumOutMax=[]  ReciprocalOutMin=[]  ReciprocalOutMax=[]  DivideOutMin=[]  DivideOutMax=[]  TunerSelectOption=Transfer Function Based (PID Tuner App)
  cfblk5 : simulink/Discrete/Tapped Delay  vinit=0.0  samptime=-1  NumDelays=1  DelayOrder=Oldest  includeCurrent=off
  cfblk6 : simulink/Discrete/Tapped Delay  vinit=0.0  samptime=-1  NumDelays=1  DelayOrder=Oldest  includeCurrent=off
  cfblk7 : simulink/Discrete/Transfer Fcn First Order  PoleZ=0.95  ICPrevOutput=0.0  DoSatur=off
      settings: SourceProductName=Simulink
  cfblk8 : Delay  DelayLengthSource=Input port
      settings: InputPortMap=u0,p1
  cfblk9 : simulink/Discrete/Transfer Fcn Lead or Lag  PoleZ=0.95  ZeroZ=0.75  ICPrevOutput=0.0  ICPrevInput=0.0  DoSatur=off
      settings: SourceProductName=Simulink  SourceProductBaseCode=SL
  cyemi_{1304..1310,1316..1317,1328..1330,1348,1361..1375} (28 alike) : DataTypeConversion  OutDataTypeStr=double
  cfblk2 : Outport
  cfblk13 : Outport  Port=2
  cfblk14 : Outport  Port=3
  wires:
  cfblk10/1 -> cyemi_1329/1, cyemi_1361/1, cyemi_1367/1, cyemi_1369/1
  cfblk1/1 -> cfblk13/1, cyemi_1317/1
  cfblk16/1(cfblk2) -> cyemi_1304/1, cyemi_1309/1
  cfblk7/1 -> cyemi_1364/1, cyemi_1373/1
  cfblk15/1(cfblk2) -> cfblk2/1, cyemi_1363/1, cyemi_1374/1
  cfblk6/1 -> cfblk14/1
  cfblk8/1 -> cyemi_1330/1, cyemi_1371/1
  cfblk3/1 -> cyemi_1365/1, cyemi_1366/1
  cfblk11/1 -> cfblk15/Action
  cfblk11/2 -> cfblk16/Action
  cfblk12/1 -> cfblk17/Action
  cfblk12/2 -> cfblk18/Action
  cyemi_1304/1 -> cfblk10/1
  cyemi_1305/1 -> cfblk11/1
  cfblk20/1 -> cyemi_1305/1
  cyemi_1306/1 -> cfblk12/1
  cfblk22/1 -> cyemi_1306/1
  cyemi_1307/1 -> cfblk15/1(cfblk1)
  cfblk19/1 -> cyemi_1307/1
  cyemi_1308/1 -> cfblk15/2(cfblk7)
  cfblk24/1 -> cyemi_1308/1
  cyemi_1309/1 -> cfblk15/3(cfblk8)
  cyemi_1310/1 -> cfblk15/4(cfblk9)
  cfblk25/1 -> cyemi_1310/1
  cyemi_1316/1 -> cfblk16/1(cfblk1)
  cfblk21/1 -> cyemi_1316/1
  cyemi_1317/1 -> cfblk16/2(cfblk10)
  cyemi_1328/1 -> cfblk17/1(cfblk1)
  cfblk23/1 -> cyemi_1328/1
  cyemi_1329/1 -> cfblk17/2(cfblk14)
  cyemi_1330/1 -> cfblk17/3(cfblk15)
  cyemi_1348/1 -> cfblk18/1(cfblk1)
  cfblk4/1 -> cyemi_1348/1
  cyemi_1361/1 -> cfblk19/1
  cyemi_1362/1 -> cfblk20/1
  cfblk17/1(cfblk2) -> cyemi_1362/1
  cyemi_1363/1 -> cfblk21/1
  cyemi_1364/1 -> cfblk22/1
  cyemi_1365/1 -> cfblk23/1
  cyemi_1366/1 -> cfblk24/1
  cyemi_1367/1 -> cfblk25/1
  cyemi_1368/1 -> cfblk3/1
  cfblk18/2(cfblk14) -> cyemi_1368/1
  cyemi_1369/1 -> cfblk4/1
  cyemi_1370/1 -> cfblk5/1
  cfblk9/1 -> cyemi_1370/1
  cyemi_1371/1 -> cfblk6/1
  cyemi_1372/1 -> cfblk7/1
  cfblk5/1 -> cyemi_1372/1
  cyemi_1373/1 -> cfblk8/1
  cyemi_1374/1 -> cfblk8/2
  cyemi_1375/1 -> cfblk9/1
  cfblk18/1(cfblk2) -> cyemi_1375/1

== system equivalent/cfblk331 ==
  cfblk1 : Inport
  cfblk9 : Inport  Port=2
  Action Port : ActionPort  ActionType=then
  cfblk13 : Subsystem  TreatAsAtomicUnit=on
  cfblk14 : Subsystem  TreatAsAtomicUnit=on
  cfblk15 : Delay
  cfblk16 : Delay
  cfblk17 : Delay
  cfblk3 : simulink/Continuous/PID Controller (2DOF)  Controller=PID  TimeDomain=Discrete-time  SampleTime=-1  IntegratorMethod=Forward Euler  FilterMethod=Forward Euler  Form=Parallel  UseFilter=on  ControllerParametersSource=internal  P=1  I=1  D=0  N=100  b=1  c=1  InitialConditionSource=internal  InitialConditionForIntegrator=0  InitialConditionForFilter=0  ExternalReset=none  LimitOutput=off  UpperSaturationLimit=inf  LowerSaturationLimit=-inf  LinearizeAsGain=off  AntiWindupMode=none  Kb=1  TrackingMode=off  Kt=1  PParamMin=[]  PParamMax=[]  IParamMin=[]  IParamMax=[]  DParamMin=[]  DParamMax=[]  NParamMin=[]  NParamMax=[]  bParamMin=[]  bParamMax=[]  cParamMin=[]  cParamMax=[]  KbParamMin=[]  KbParamMax=[]  KtParamMin=[]  KtParamMax=[]  POutMin=[]  POutMax=[]  IOutMin=[]  IOutMax=[]  DOutMin=[]  DOutMax=[]  NOutMin=[]  NOutMax=[]  bOutMin=[]  bOutMax=[]  cOutMin=[]  cOutMax=[]  KbOutMin=[]  KbOutMax=[]  KtOutMin=[]  KtOutMax=[]  IntegratorOutMin=[]  IntegratorOutMax=[]  FilterOutMin=[]  FilterOutMax=[]  SumOutMin=[]  SumOutMax=[]  Sum1OutMin=[]  Sum1OutMax=[]  Sum2OutMin=[]  Sum2OutMax=[]  Sum3OutMin=[]  Sum3OutMax=[]  SumI1OutMin=[]  SumI1OutMax=[]  SumI2OutMin=[]  SumI2OutMax=[]  SumI3OutMin=[]  SumI3OutMax=[]  SumDOutMin=[]  SumDOutMax=[]  SaturationOutMin=[]  SaturationOutMax=[]  IntegratorContinuousStateAttributes=''  IntegratorStateMustResolveToSignalObject=off  IntegratorRTWStateStorageClass=Auto  FilterContinuousStateAttributes=''  FilterStateMustResolveToSignalObject=off  FilterRTWStateStorageClass=Auto  DifferentiatorICPrevScaledInput=0  DifferentiatorOutMin=[]  DifferentiatorOutMax=[]  FilterDiffOutCoefMin=[]  FilterDiffOutCoefMax=[]  SumDenOutMin=[]  SumDenOutMax=[]  SumNumOutMin=[]  SumNumOutMax=[]  ReciprocalOutMin=[]  ReciprocalOutMax=[]  DivideOutMin=[]  DivideOutMax=[]  TunerSelectOption=Transfer Function Based (PID Tuner App)
  cfblk4 : DiscreteFilter
  cfblk5 : simulink/Discrete/Transfer Fcn Real Zero  ZeroZ=0.75  ICPrevInput=0.0  DoSatur=off
      settings: SourceProductName=Simulink  SourceProductBaseCode=SL
  cfblk6 : DiscreteZeroPole  Poles=[0 0.5]  Gain=1  SampleTime=-1
  cfblk7 : simulink/Continuous/PID Controller  Controller=PID  TimeDomain=Discrete-time  SampleTime=-1  IntegratorMethod=Forward Euler  FilterMethod=Forward Euler  Form=Parallel  UseFilter=on  ControllerParametersSource=internal  P=1  I=1  D=0  N=100  InitialConditionSource=internal  InitialConditionForIntegrator=0  InitialConditionForFilter=0  ExternalReset=none  LimitOutput=off  UpperSaturationLimit=inf  LowerSaturationLimit=-inf  LinearizeAsGain=off  AntiWindupMode=none  Kb=1  TrackingMode=off  Kt=1  PParamMin=[]  PParamMax=[]  IParamMin=[]  IParamMax=[]  DParamMin=[]  DParamMax=[]  NParamMin=[]  NParamMax=[]  KbParamMin=[]  KbParamMax=[]  KtParamMin=[]  KtParamMax=[]  POutMin=[]  POutMax=[]  IOutMin=[]  IOutMax=[]  DOutMin=[]  DOutMax=[]  NOutMin=[]  NOutMax=[]  KbOutMin=[]  KbOutMax=[]  KtOutMin=[]  KtOutMax=[]  IntegratorOutMin=[]  IntegratorOutMax=[]  FilterOutMin=[]  FilterOutMax=[]  SumOutMin=[]  SumOutMax=[]  SumI1OutMin=[]  SumI1OutMax=[]  SumI2OutMin=[]  SumI2OutMax=[]  SumI3OutMin=[]  SumI3OutMax=[]  SumDOutMin=[]  SumDOutMax=[]  SaturationOutMin=[]  SaturationOutMax=[]  IntegratorContinuousStateAttributes=''  IntegratorStateMustResolveToSignalObject=off  IntegratorRTWStateStorageClass=Auto  FilterContinuousStateAttributes=''  FilterStateMustResolveToSignalObject=off  FilterRTWStateStorageClass=Auto  DifferentiatorICPrevScaledInput=0  DifferentiatorOutMin=[]  DifferentiatorOutMax=[]  FilterDiffOutCoefMin=[]  FilterDiffOutCoefMax=[]  SumDenOutMin=[]  SumDenOutMax=[]  SumNumOutMin=[]  SumNumOutMax=[]  ReciprocalOutMin=[]  ReciprocalOutMax=[]  DivideOutMin=[]  DivideOutMax=[]  TunerSelectOption=Transfer Function Based (PID Tuner App)
  cfblk8 : If  SampleTime=1
  cyemi_{1378..1381,1393..1396,1404..1413} (18 alike) : DataTypeConversion  OutDataTypeStr=double
  cfblk2 : Outport
  cfblk10 : Outport  Port=2
  cfblk11 : Outport  Port=3
  cfblk12 : Outport  Port=4
  wires:
  cfblk7/1 -> cyemi_1380/1, cyemi_1381/1, cyemi_1413/1
  cfblk4/1 -> cfblk12/1, cyemi_1404/1, cyemi_1406/1
  cfblk6/1 -> cfblk10/1
  cfblk1/1 -> cyemi_1394/1, cyemi_1396/1, cyemi_1407/1, cyemi_1410/1
  cfblk9/1 -> cfblk11/1
  cfblk14/1(cfblk2) -> cfblk2/1
  cfblk3/1 -> cyemi_1379/1, cyemi_1395/1, cyemi_1412/1
  cfblk8/1 -> cfblk13/Action
  cfblk8/2 -> cfblk14/Action
  cyemi_1378/1 -> cfblk13/1(cfblk1)
  cfblk16/1 -> cyemi_1378/1
  cyemi_1379/1 -> cfblk13/2(cfblk11)
  cyemi_1380/1 -> cfblk13/3(cfblk12)
  cyemi_1381/1 -> cfblk13/4(cfblk13)
  cyemi_1393/1 -> cfblk14/1(cfblk1)
  cfblk15/1 -> cyemi_1393/1
  cyemi_1394/1 -> cfblk14/2(cfblk10)
  cyemi_1395/1 -> cfblk14/3(cfblk11)
  cyemi_1396/1 -> cfblk14/4(cfblk12)
  cyemi_1404/1 -> cfblk15/1
  cyemi_1405/1 -> cfblk16/1
  cfblk14/2(cfblk13) -> cyemi_1405/1
  cyemi_1406/1 -> cfblk17/1
  cyemi_1407/1 -> cfblk3/1
  cyemi_1408/1 -> cfblk3/2
  cfblk17/1 -> cyemi_1408/1
  cyemi_1409/1 -> cfblk4/1
  cfblk13/1(cfblk2) -> cyemi_1409/1
  cyemi_1410/1 -> cfblk5/1
  cyemi_1411/1 -> cfblk6/1
  cfblk5/1 -> cyemi_1411/1
  cyemi_1412/1 -> cfblk7/1
  cyemi_1413/1 -> cfblk8/1

== system equivalent/cfblk332 ==
  cfblk1 : Inport
  cfblk9 : Inport  Port=2
  Action Port : ActionPort  ActionType=else
  cfblk13 : Delay
  cfblk3 : simulink/Discrete/Tapped Delay  vinit=0.0  samptime=-1  NumDelays=1  DelayOrder=Oldest  includeCurrent=off
  cfblk4 : simulink/Continuous/PID Controller  Controller=PID  TimeDomain=Discrete-time  SampleTime=-1  IntegratorMethod=Forward Euler  FilterMethod=Forward Euler  Form=Parallel  UseFilter=on  ControllerParametersSource=internal  P=1  I=1  D=0  N=100  InitialConditionSource=internal  InitialConditionForIntegrator=0  InitialConditionForFilter=0  ExternalReset=none  LimitOutput=off  UpperSaturationLimit=inf  LowerSaturationLimit=-inf  LinearizeAsGain=off  AntiWindupMode=none  Kb=1  TrackingMode=off  Kt=1  PParamMin=[]  PParamMax=[]  IParamMin=[]  IParamMax=[]  DParamMin=[]  DParamMax=[]  NParamMin=[]  NParamMax=[]  KbParamMin=[]  KbParamMax=[]  KtParamMin=[]  KtParamMax=[]  POutMin=[]  POutMax=[]  IOutMin=[]  IOutMax=[]  DOutMin=[]  DOutMax=[]  NOutMin=[]  NOutMax=[]  KbOutMin=[]  KbOutMax=[]  KtOutMin=[]  KtOutMax=[]  IntegratorOutMin=[]  IntegratorOutMax=[]  FilterOutMin=[]  FilterOutMax=[]  SumOutMin=[]  SumOutMax=[]  SumI1OutMin=[]  SumI1OutMax=[]  SumI2OutMin=[]  SumI2OutMax=[]  SumI3OutMin=[]  SumI3OutMax=[]  SumDOutMin=[]  SumDOutMax=[]  SaturationOutMin=[]  SaturationOutMax=[]  IntegratorContinuousStateAttributes=''  IntegratorStateMustResolveToSignalObject=off  IntegratorRTWStateStorageClass=Auto  FilterContinuousStateAttributes=''  FilterStateMustResolveToSignalObject=off  FilterRTWStateStorageClass=Auto  DifferentiatorICPrevScaledInput=0  DifferentiatorOutMin=[]  DifferentiatorOutMax=[]  FilterDiffOutCoefMin=[]  FilterDiffOutCoefMax=[]  SumDenOutMin=[]  SumDenOutMax=[]  SumNumOutMin=[]  SumNumOutMax=[]  ReciprocalOutMin=[]  ReciprocalOutMax=[]  DivideOutMin=[]  DivideOutMax=[]  TunerSelectOption=Transfer Function Based (PID Tuner App)
  cfblk5 : DiscreteTransferFcn
  cfblk6 : simulink/Discrete/Difference  ICPrevInput=0.0  OutMin=[]  OutMax=[]  OutDataTypeStr=Inherit: Inherit via back propagation  OutDataType=fixdt(1, 16)  OutScaling=2^-10  DoSatur=off
  cfblk7 : simulink/Discrete/Transfer Fcn First Order  PoleZ=0.95  ICPrevOutput=0.0  DoSatur=off
      settings: SourceProductName=Simulink
  cfblk8 : UnitDelay  SampleTime=-1
  cyemi_{1416..1422} (7 alike) : DataTypeConversion  OutDataTypeStr=double
  cfblk2 : Outport
  cfblk10 : Outport  Port=2
  cfblk11 : Outport  Port=3
  cfblk12 : Outport  Port=4
  wires:
  cfblk3/1 -> cyemi_1418/1, cyemi_1422/1
  cfblk8/1 -> cfblk12/1, cfblk10/1
  cfblk9/1 -> cfblk11/1
  cfblk5/1 -> cfblk2/1
  cyemi_1416/1 -> cfblk13/1
  cfblk4/1 -> cyemi_1416/1
  cyemi_1417/1 -> cfblk3/1
  cfblk13/1 -> cyemi_1417/1
  cyemi_1418/1 -> cfblk4/1
  cyemi_1419/1 -> cfblk5/1
  cfblk6/1 -> cyemi_1419/1
  cyemi_1420/1 -> cfblk6/1
  cfblk7/1 -> cyemi_1420/1
  cyemi_1421/1 -> cfblk7/1
  cfblk1/1 -> cyemi_1421/1
  cyemi_1422/1 -> cfblk8/1

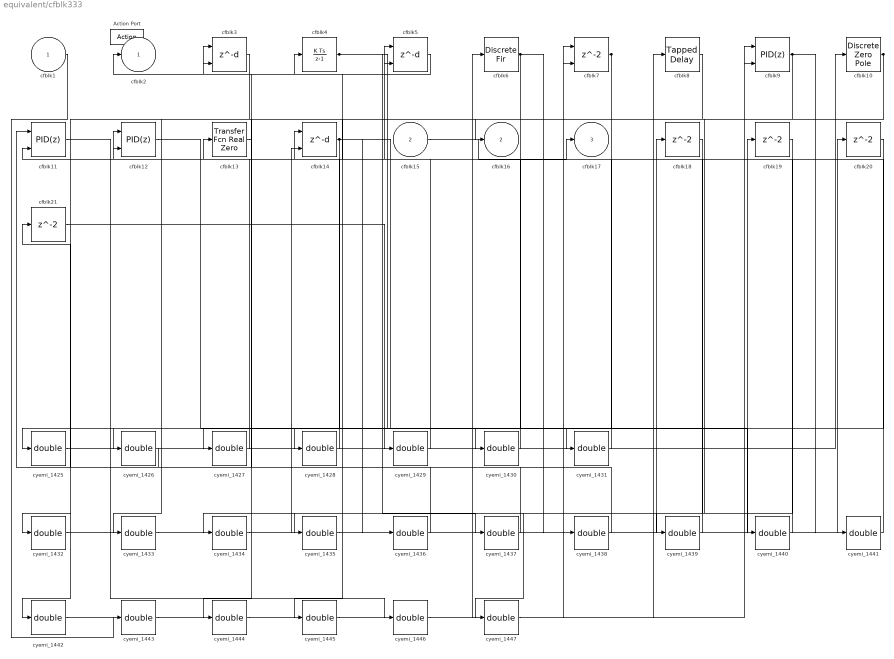
== system equivalent/cfblk333 ==
  cfblk1 : Inport
  cfblk15 : Inport  Port=2
  Action Port : ActionPort  ActionType=then
  cfblk10 : DiscreteZeroPole  Poles=[0 0.5]  Gain=1  SampleTime=-1
  cfblk11 : simulink/Continuous/PID Controller (2DOF)  Controller=PID  TimeDomain=Discrete-time  SampleTime=-1  IntegratorMethod=Forward Euler  FilterMethod=Forward Euler  Form=Parallel  UseFilter=on  ControllerParametersSource=internal  P=1  I=1  D=0  N=100  b=1  c=1  InitialConditionSource=internal  InitialConditionForIntegrator=0  InitialConditionForFilter=0  ExternalReset=none  LimitOutput=off  UpperSaturationLimit=inf  LowerSaturationLimit=-inf  LinearizeAsGain=off  AntiWindupMode=none  Kb=1  TrackingMode=off  Kt=1  PParamMin=[]  PParamMax=[]  IParamMin=[]  IParamMax=[]  DParamMin=[]  DParamMax=[]  NParamMin=[]  NParamMax=[]  bParamMin=[]  bParamMax=[]  cParamMin=[]  cParamMax=[]  KbParamMin=[]  KbParamMax=[]  KtParamMin=[]  KtParamMax=[]  POutMin=[]  POutMax=[]  IOutMin=[]  IOutMax=[]  DOutMin=[]  DOutMax=[]  NOutMin=[]  NOutMax=[]  bOutMin=[]  bOutMax=[]  cOutMin=[]  cOutMax=[]  KbOutMin=[]  KbOutMax=[]  KtOutMin=[]  KtOutMax=[]  IntegratorOutMin=[]  IntegratorOutMax=[]  FilterOutMin=[]  FilterOutMax=[]  SumOutMin=[]  SumOutMax=[]  Sum1OutMin=[]  Sum1OutMax=[]  Sum2OutMin=[]  Sum2OutMax=[]  Sum3OutMin=[]  Sum3OutMax=[]  SumI1OutMin=[]  SumI1OutMax=[]  SumI2OutMin=[]  SumI2OutMax=[]  SumI3OutMin=[]  SumI3OutMax=[]  SumDOutMin=[]  SumDOutMax=[]  SaturationOutMin=[]  SaturationOutMax=[]  IntegratorContinuousStateAttributes=''  IntegratorStateMustResolveToSignalObject=off  IntegratorRTWStateStorageClass=Auto  FilterContinuousStateAttributes=''  FilterStateMustResolveToSignalObject=off  FilterRTWStateStorageClass=Auto  DifferentiatorICPrevScaledInput=0  DifferentiatorOutMin=[]  DifferentiatorOutMax=[]  FilterDiffOutCoefMin=[]  FilterDiffOutCoefMax=[]  SumDenOutMin=[]  SumDenOutMax=[]  SumNumOutMin=[]  SumNumOutMax=[]  ReciprocalOutMin=[]  ReciprocalOutMax=[]  DivideOutMin=[]  DivideOutMax=[]  TunerSelectOption=Transfer Function Based (PID Tuner App)
  cfblk12 : simulink/Continuous/PID Controller (2DOF)  Controller=PID  TimeDomain=Discrete-time  SampleTime=-1  IntegratorMethod=Forward Euler  FilterMethod=Forward Euler  Form=Parallel  UseFilter=on  ControllerParametersSource=internal  P=1  I=1  D=0  N=100  b=1  c=1  InitialConditionSource=internal  InitialConditionForIntegrator=0  InitialConditionForFilter=0  ExternalReset=none  LimitOutput=off  UpperSaturationLimit=inf  LowerSaturationLimit=-inf  LinearizeAsGain=off  AntiWindupMode=none  Kb=1  TrackingMode=off  Kt=1  PParamMin=[]  PParamMax=[]  IParamMin=[]  IParamMax=[]  DParamMin=[]  DParamMax=[]  NParamMin=[]  NParamMax=[]  bParamMin=[]  bParamMax=[]  cParamMin=[]  cParamMax=[]  KbParamMin=[]  KbParamMax=[]  KtParamMin=[]  KtParamMax=[]  POutMin=[]  POutMax=[]  IOutMin=[]  IOutMax=[]  DOutMin=[]  DOutMax=[]  NOutMin=[]  NOutMax=[]  bOutMin=[]  bOutMax=[]  cOutMin=[]  cOutMax=[]  KbOutMin=[]  KbOutMax=[]  KtOutMin=[]  KtOutMax=[]  IntegratorOutMin=[]  IntegratorOutMax=[]  FilterOutMin=[]  FilterOutMax=[]  SumOutMin=[]  SumOutMax=[]  Sum1OutMin=[]  Sum1OutMax=[]  Sum2OutMin=[]  Sum2OutMax=[]  Sum3OutMin=[]  Sum3OutMax=[]  SumI1OutMin=[]  SumI1OutMax=[]  SumI2OutMin=[]  SumI2OutMax=[]  SumI3OutMin=[]  SumI3OutMax=[]  SumDOutMin=[]  SumDOutMax=[]  SaturationOutMin=[]  SaturationOutMax=[]  IntegratorContinuousStateAttributes=''  IntegratorStateMustResolveToSignalObject=off  IntegratorRTWStateStorageClass=Auto  FilterContinuousStateAttributes=''  FilterStateMustResolveToSignalObject=off  FilterRTWStateStorageClass=Auto  DifferentiatorICPrevScaledInput=0  DifferentiatorOutMin=[]  DifferentiatorOutMax=[]  FilterDiffOutCoefMin=[]  FilterDiffOutCoefMax=[]  SumDenOutMin=[]  SumDenOutMax=[]  SumNumOutMin=[]  SumNumOutMax=[]  ReciprocalOutMin=[]  ReciprocalOutMax=[]  DivideOutMin=[]  DivideOutMax=[]  TunerSelectOption=Transfer Function Based (PID Tuner App)
  cfblk13 : simulink/Discrete/Transfer Fcn Real Zero  ZeroZ=0.75  ICPrevInput=0.0  DoSatur=off
      settings: SourceProductName=Simulink  SourceProductBaseCode=SL
  cfblk14 : Delay  DelayLengthSource=Input port
      settings: InputPortMap=u0,p1
  cfblk{18..21} (4 alike) : Delay
  cfblk3 : Delay  DelayLengthSource=Input port
      settings: InputPortMap=u0,p1
  cfblk4 : DiscreteIntegrator  SampleTime=-1  ICPrevOutput=DiscIntNeverNeededParam  ICPrevScaledInput=DiscIntNeverNeededParam
  cfblk5 : Delay  DelayLengthSource=Input port
      settings: InputPortMap=u0,p1
  cfblk6 : DiscreteFir
  cfblk7 : Delay  ShowEnablePort=on
      settings: InputPortMap=u0,e6
  cfblk8 : simulink/Discrete/Tapped Delay  vinit=0.0  samptime=-1  NumDelays=1  DelayOrder=Oldest  includeCurrent=off
  cfblk9 : simulink/Continuous/PID Controller (2DOF)  Controller=PID  TimeDomain=Discrete-time  SampleTime=-1  IntegratorMethod=Forward Euler  FilterMethod=Forward Euler  Form=Parallel  UseFilter=on  ControllerParametersSource=internal  P=1  I=1  D=0  N=100  b=1  c=1  InitialConditionSource=internal  InitialConditionForIntegrator=0  InitialConditionForFilter=0  ExternalReset=none  LimitOutput=off  UpperSaturationLimit=inf  LowerSaturationLimit=-inf  LinearizeAsGain=off  AntiWindupMode=none  Kb=1  TrackingMode=off  Kt=1  PParamMin=[]  PParamMax=[]  IParamMin=[]  IParamMax=[]  DParamMin=[]  DParamMax=[]  NParamMin=[]  NParamMax=[]  bParamMin=[]  bParamMax=[]  cParamMin=[]  cParamMax=[]  KbParamMin=[]  KbParamMax=[]  KtParamMin=[]  KtParamMax=[]  POutMin=[]  POutMax=[]  IOutMin=[]  IOutMax=[]  DOutMin=[]  DOutMax=[]  NOutMin=[]  NOutMax=[]  bOutMin=[]  bOutMax=[]  cOutMin=[]  cOutMax=[]  KbOutMin=[]  KbOutMax=[]  KtOutMin=[]  KtOutMax=[]  IntegratorOutMin=[]  IntegratorOutMax=[]  FilterOutMin=[]  FilterOutMax=[]  SumOutMin=[]  SumOutMax=[]  Sum1OutMin=[]  Sum1OutMax=[]  Sum2OutMin=[]  Sum2OutMax=[]  Sum3OutMin=[]  Sum3OutMax=[]  SumI1OutMin=[]  SumI1OutMax=[]  SumI2OutMin=[]  SumI2OutMax=[]  SumI3OutMin=[]  SumI3OutMax=[]  SumDOutMin=[]  SumDOutMax=[]  SaturationOutMin=[]  SaturationOutMax=[]  IntegratorContinuousStateAttributes=''  IntegratorStateMustResolveToSignalObject=off  IntegratorRTWStateStorageClass=Auto  FilterContinuousStateAttributes=''  FilterStateMustResolveToSignalObject=off  FilterRTWStateStorageClass=Auto  DifferentiatorICPrevScaledInput=0  DifferentiatorOutMin=[]  DifferentiatorOutMax=[]  FilterDiffOutCoefMin=[]  FilterDiffOutCoefMax=[]  SumDenOutMin=[]  SumDenOutMax=[]  SumNumOutMin=[]  SumNumOutMax=[]  ReciprocalOutMin=[]  ReciprocalOutMax=[]  DivideOutMin=[]  DivideOutMax=[]  TunerSelectOption=Transfer Function Based (PID Tuner App)
  cyemi_{1425..1447} (23 alike) : DataTypeConversion  OutDataTypeStr=double
  cfblk2 : Outport
  cfblk16 : Outport  Port=2
  cfblk17 : Outport  Port=3
  wires:
  cfblk6/1 -> cyemi_1435/1, cyemi_1438/1
  cfblk9/1 -> cyemi_1425/1, cyemi_1432/1, cyemi_1441/1
  cfblk15/1 -> cfblk17/1
  cfblk14/1 -> cyemi_1430/1, cyemi_1436/1, cyemi_1442/1
  cfblk10/1 -> cyemi_1428/1, cyemi_1439/1
  cfblk7/1 -> cfblk16/1, cyemi_1445/1
  cfblk4/1 -> cyemi_1437/1, cyemi_1440/1
  cfblk5/1 -> cfblk2/1
  cyemi_1425/1 -> cfblk10/1
  cyemi_1426/1 -> cfblk11/1
  cfblk20/1 -> cyemi_1426/1
  cyemi_1427/1 -> cfblk11/2
  cfblk8/1 -> cyemi_1427/1
  cyemi_1428/1 -> cfblk12/1
  cyemi_1429/1 -> cfblk12/2
  cfblk21/1 -> cyemi_1429/1
  cyemi_1430/1 -> cfblk13/1
  cyemi_1431/1 -> cfblk14/1
  cfblk12/1 -> cyemi_1431/1
  cyemi_1432/1 -> cfblk14/2
  cyemi_1433/1 -> cfblk18/1
  cfblk3/1 -> cyemi_1433/1
  cyemi_1434/1 -> cfblk19/1
  cfblk13/1 -> cyemi_1434/1
  cyemi_1435/1 -> cfblk20/1
  cyemi_1436/1 -> cfblk21/1
  cyemi_1437/1 -> cfblk3/1
  cyemi_1438/1 -> cfblk3/2
  cyemi_1439/1 -> cfblk4/1
  cyemi_1440/1 -> cfblk5/1
  cyemi_1441/1 -> cfblk5/2
  cyemi_1442/1 -> cfblk6/1
  cyemi_1443/1 -> cfblk7/1
  cfblk1/1 -> cyemi_1443/1
  cyemi_1444/1 -> cfblk7/2
  cfblk19/1 -> cyemi_1444/1
  cyemi_1445/1 -> cfblk8/1
  cyemi_1446/1 -> cfblk9/1
  cfblk11/1 -> cyemi_1446/1
  cyemi_1447/1 -> cfblk9/2
  cfblk18/1 -> cyemi_1447/1

== system equivalent/cfblk334 ==
  cfblk1 : Inport
  cfblk6 : Inport  Port=2
  Action Port : ActionPort  ActionType=else
  cfblk10 : Delay
  cfblk11 : Delay
  cfblk3 : DiscreteIntegrator  SampleTime=-1  ICPrevOutput=DiscIntNeverNeededParam  ICPrevScaledInput=DiscIntNeverNeededParam
  cfblk4 : UnitDelay  SampleTime=-1
  cfblk5 : If  SampleTime=1
  cfblk8 : Subsystem  TreatAsAtomicUnit=on
  cfblk9 : Subsystem  TreatAsAtomicUnit=on
  cyemi_{1450..1456,1461..1462} (9 alike) : DataTypeConversion  OutDataTypeStr=double
  cfblk2 : Outport
  cfblk7 : Outport  Port=2
  wires:
  cfblk4/1 -> cfblk7/1
  cfblk8/3(cfblk9) -> cfblk2/1
  cfblk5/1 -> cfblk8/Action
  cfblk5/2 -> cfblk9/Action
  cyemi_1450/1 -> cfblk10/1
  cfblk9/1(cfblk2) -> cyemi_1450/1
  cyemi_1451/1 -> cfblk11/1
  cfblk9/2(cfblk10) -> cyemi_1451/1
  cyemi_1452/1 -> cfblk3/1
  cfblk6/1 -> cyemi_1452/1
  cyemi_1453/1 -> cfblk4/1
  cfblk3/1 -> cyemi_1453/1
  cyemi_1454/1 -> cfblk5/1
  cfblk1/1 -> cyemi_1454/1
  cyemi_1455/1 -> cfblk8/1(cfblk1)
  cfblk10/1 -> cyemi_1455/1
  cyemi_1456/1 -> cfblk8/2(cfblk7)
  cfblk11/1 -> cyemi_1456/1
  cyemi_1461/1 -> cfblk9/1(cfblk1)
  cfblk8/1(cfblk2) -> cyemi_1461/1
  cyemi_1462/1 -> cfblk9/2(cfblk9)
  cfblk8/2(cfblk8) -> cyemi_1462/1
